simulink model "fmcw_chirp_rom_test"  (R2025b)
settings: Solver=FixedStepDiscrete  StartTime=0.0  StopTime=1.024e-05  FixedStep=5e-09  RelTol=1e-3
libraries: simulink x1
settings Model: DataTypeOverride=Off  Creator=kimsteph  LastModifiedBy=kimsteph
settings OptimizationCC: BlockReduction=off  ConditionallyExecuteInputs=off  DefaultParameterBehavior=Inlined  InheritOutputTypeSmallerThanSingle=on
settings DebuggingCC: ArtificialAlgebraicLoopMsg=error  SingleTaskRateTransMsg=error
settings HardwareCC: ProdBitPerPointer=32.0  ProdBitPerSizeT=32.0  ProdBitPerPtrDiffT=32.0  ProdLargestAtomicFloat=None  ProdIntDivRoundTo=Undefined  ProdEndianess=Unspecified  ProdWordSize=32.0  ProdHWDeviceType=ASIC/FPGA->ASIC/FPGA  TargetBitPerPointer=64.0  TargetBitPerSizeT=64.0  TargetBitPerPtrDiffT=64.0  TargetLongLongMode=on  TargetIntDivRoundTo=Zero  TargetEndianess=LittleEndian  TargetWordSize=64.0  TargetHWDeviceType=Custom Processor->MATLAB Host Computer  ProdEqTarget=off

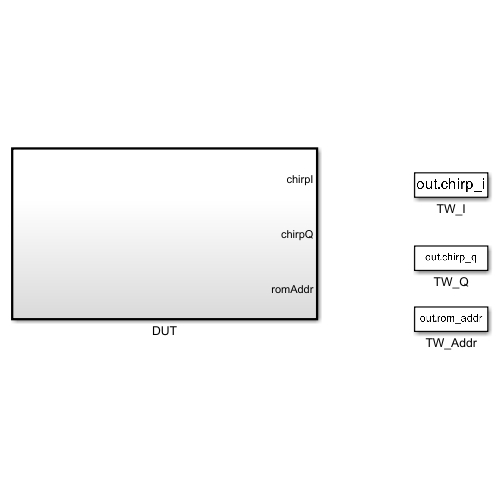
[thumbnail: Simulink's stored preview of the top-level diagram]
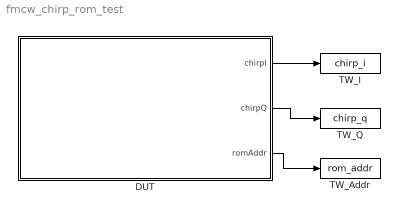
== system fmcw_chirp_rom_test ==
  DUT : Subsystem  TreatAsAtomicUnit=on
  TW_Addr : ToWorkspace  VariableName=rom_addr  SaveFormat=Timeseries  SampleTime=-1
  TW_I : ToWorkspace  VariableName=chirp_i  SaveFormat=Timeseries  SampleTime=-1
  TW_Q : ToWorkspace  VariableName=chirp_q  SaveFormat=Timeseries  SampleTime=-1
  wires:
  DUT/2(chirpQ) -> TW_Q/1
  DUT/1(chirpI) -> TW_I/1
  DUT/3(romAddr) -> TW_Addr/1

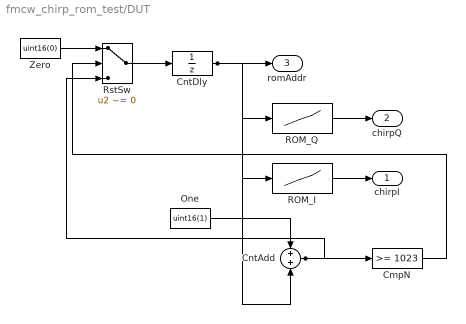
== system fmcw_chirp_rom_test/DUT ==
  CmpN : simulink/Logic and Bit Operations/Compare To Constant  relop=>=  const=1023  OutDataTypeStr=boolean
  CntAdd : Sum  OutDataTypeStr=uint16
  CntDly : UnitDelay  SampleTime=5e-09  HasFrameUpgradeWarning=on
  One : Constant  Value=uint16(1)  OutDataTypeStr=uint16
  ROM_I : Lookup_n-D  NumberOfTableDimensions=1  BreakpointsForDimension1=[0 1 2 3 4 5 6 7 8 9 10 11 12 13 14 15 16 17 18 19 20 21 22 23 24 25 26 27 28 29 30 31 32 33 34 35 36 37 38 39 40 41 42 43 44 45 46 47 48 49 50 51 52 53 54 55 56 57 58 59 60 61 62 63 64 65 66 67 68 69 70 71 72 73 74 75 76 77 78 79 80 81 82 83 84 85 86 87 88 89 90 91 92 93 94 95 96 97 98 99 100 101 102 103 104 105 106 107 108 109 110 111 112 113 114 115 116 117 118 119 120 121 122 123 124 125 126 127 128 129 130 131 132 133 134 135 136 137 138 139 140 141 142 143 144 145 146 147 148 149 150 151 152 153 154 155 156 157 158 159 160 161 162 163 164 165 166 167 168 169 170 171 172 173 174 175 176 177 178 179 180 181 182 183 184 185 186 187 188 189 190 191 192 193 194 195 196 197 198 199 200 201 202 203 204 205 206 207 208 209 210 211 212 213 214 215 216 217 218 219 220 221 222 223 224 225 226 227 228 229 230 231 232 233 234 235 236 237 238 239 240 241 242 243 244 245 246 247 248 249 250 251 252 253 254 255 256 257 258 259 260 261 262 263 264 265 266 267 268 269 270 271 272 273 274 275 276 277 278 279 280 281 282 283 284 285 286 287 288 289 290 291 292 293 294 295 296 297 298 299 300 301 302 303 304 305 306 307 308 309 310 311 312 313 314 315 316 317 318 319 320 321 322 323 324 325 326 327 328 329 330 331 332 333 334 335 336 337 338 339 340 341 342 343 344 345 346 347 348 349 350 351 352 353 354 355 356 357 358 359 360 361 362 363 364 365 366 367 368 369 370 371 372 373 374 375 376 377 378 379 380 381 382 383 384 385 386 387 388 389 390 391 392 393 394 395 396 397 398 399 400 401 402 403 404 405 406 407 408 409 410 411 412 413 414 415 416 417 418 419 420 421 422 423 424 425 426 427 428 429 430 431 432 433 434 435 436 437 438 439 440 441 442 443 444 445 446 447 448 449 450 451 452 453 454 455 456 457 458 459 460 461 462 463 464 465 466 467 468 469 470 471 472 473 474 475 476 477 478 479 480 481 482 483 484 485 486 487 488 489 490 491 492 493 494 495 496 497 498 499 500 501 502 503 504 505 506 507 508 509 510 511 512 513 514 515 516 517 518 519 520 521 522 523 524 525 526 527 528 529 530 531 532 533 534 535 536 537 538 539 540 541 542 543 544 545 546 547 548 549 550 551 552 553 554 555 556 557 558 559 560 561 562 563 564 565 566 567 568 569 570 571 572 573 574 575 576 577 578 579 580 581 582 583 584 585 586 587 588 589 590 591 592 593 594 595 596 597 598 599 600 601 602 603 604 605 606 607 608 609 610 611 612 613 614 615 616 617 618 619 620 621 622 623 624 625 626 627 628 629 630 631 632 633 634 635 636 637 638 639 640 641 642 643 644 645 646 647 648 649 650 651 652 653 654 655 656 657 658 659 660 661 662 663 664 665 666 667 668 669 670 671 672 673 674 675 676 677 678 679 680 681 682 683 684 685 686 687 688 689 690 691 692 693 694 695 696 697 698 699 700 701 702 703 704 705 706 707 708 709 710 711 712 713 714 715 716 717 718 719 720 721 722 723 724 725 726 727 728 729 730 731 732 733 734 735 736 737 738 739 740 741 742 743 744 745 746 747 748 749 750 751 752 753 754 755 756 757 758 759 760 761 762 763 764 765 766 767 768 769 770 771 772 773 774 775 776 777 778 779 780 781 782 783 784 785 786 787 788 789 790 791 792 793 794 795 796 797 798 799 800 801 802 803 804 805 806 807 808 809 810 811 812 813 814 815 816 817 818 819 820 821 822 823 824 825 826 827 828 829 830 831 832 833 834 835 836 837 838 839 840 841 842 843 844 845 846 847 848 849 850 851 852 853 854 855 856 857 858 859 860 861 862 863 864 865 866 867 868 869 870 871 872 873 874 875 876 877 878 879 880 881 882 883 884 885 886 887 888 889 890 891 892 893 894 895 896 897 898 899 900 901 902 903 904 905 906 907 908 909 910 911 912 913 914 915 916 917 918 919 920 921 922 923 924 925 926 927 928 929 930 931 932 933 934 935 936 937 938 939 940 941 942 943 944 945 946 947 948 949 950 951 952 953 954 955 956 957 958 959 960 961 962 963 964 965 966 967 968 969 970 971 972 973 974 975 976 977 978 979 980 981 982 983 984 985 986 987 988 989 990 991 992 993 994 995 996 997 998 999 1000 1001 1002 1003 1004 1005 1006 1007 1008 1009 1010 1011 1012 1013 1014 1015 1016 1017 1018 1019 1020 1021 1022 1023]  Table=[1;0.999999;0.999981;0.999905;0.999699;0.999265;0.998476;0.997176;0.995185;0.992291;0.988258;0.982824;0.975702;0.966584;0.955141;0.941026;0.92388;0.903332;0.879012;0.850549;0.817585;0.779778;0.736817;0.688429;0.634393;0.574553;0.50883;0.437237;0.359895;0.277046;0.189069;0.0964904;-1.60812e-16;-0.0995436;-0.201105;-0.303468;-0.405241;-0.504863;-0.600616;-0.690651;-0.77301;-0.845673;-0.906596;-0.953768;-0.985278;-0.999378;-0.994565;-0.969657;-0.92388;-0.856939;-0.769103;-0.661266;-0.534998;-0.392582;-0.237024;-0.0720347;0.0980171;0.268191;0.433094;0.58704;0.724247;0.83906;0.92621;0.981083;1;0.980485;0.921514;0.823721;0.689541;0.523283;0.331106;0.120888;-0.0980171;-0.315138;-0.519356;-0.699473;-0.844854;-0.946105;-0.995767;-0.98895;-0.92388;-0.802293;-0.629638;-0.415034;-0.170962;0.0873255;0.342661;0.577062;0.77301;0.91483;0.990058;0.990695;0.91421;0.764179;0.550458;0.288816;2.32745e-15;-0.291752;-0.560662;-0.781695;-0.932993;-0.998211;-0.968522;-0.844032;-0.634393;-0.358463;-0.0429383;0.279993;0.575808;0.811355;0.958703;0.998719;0.92388;0.73992;0.465976;0.133061;-0.219101;-0.54661;-0.806848;-0.964184;-0.995185;-0.892534;-0.667;-0.34698;0.0245412;0.395401;0.711432;0.924465;1;0.923291;0.702755;0.369892;-0.0245412;-0.417824;-0.745058;-0.950008;-0.995185;-0.86933;-0.59076;-0.20561;0.219101;0.606731;0.884797;0.99887;0.92388;0.670422;0.284408;-0.160372;-0.575808;-0.876809;-0.999078;-0.913587;-0.634393;-0.217604;0.248928;0.663564;0.932993;0.993737;0.828045;0.470043;6.85988e-15;-0.472749;-0.834863;-0.996443;-0.91421;-0.60429;-0.140658;0.361326;0.77301;0.985539;0.939459;0.642657;0.170962;-0.349856;-0.776888;-0.9894;-0.92388;-0.594466;-0.091909;0.439994;0.844854;0.999942;0.854558;0.448241;-0.0980171;-0.61644;-0.943593;-0.972584;-0.689541;-0.181532;0.388345;0.832321;1;0.830616;0.377007;-0.208612;-0.724247;-0.987544;-0.901349;-0.491563;0.0980171;0.654334;0.971504;0.927935;0.534998;-0.0628518;-0.639124;-0.970403;-0.92388;-0.512786;0.104122;0.681724;0.985278;0.886932;0.422;-0.220598;-0.77301;-0.999735;-0.799537;-0.253382;0.405241;0.888345;0.97957;0.633207;-5.8814e-15;-0.635578;-0.981964;-0.875329;-0.359895;0.32676;0.860867;0.985014;0.634393;-0.0260747;-0.676093;-0.994075;-0.817585;-0.229565;0.476799;0.94206;0.92388;0.426168;-0.296151;-0.864744;-0.975702;-0.564466;0.152797;0.789289;0.995185;0.652011;-0.0551952;-0.733697;-0.999699;-0.697278;0.00613588;0.708191;1;0.706021;-0.00613588;-0.716801;-0.999699;-0.679476;0.0551952;0.75821;0.995185;0.614022;-0.152797;-0.825456;-0.975702;-0.502212;0.296151;0.904644;0.92388;0.335445;-0.476799;-0.973293;-0.817585;-0.108697;0.676093;0.99966;0.634393;-0.172473;-0.860867;-0.945107;-0.359895;0.483527;0.981964;0.772036;1.02889e-14;-0.773983;-0.97957;-0.459177;0.405241;0.967366;0.799537;0.0230077;-0.77301;-0.975365;-0.422;0.4619;0.985278;0.731609;-0.104122;-0.858516;-0.92388;-0.241492;0.639124;0.998023;0.534998;-0.372741;-0.971504;-0.756206;0.0980171;0.870842;0.901349;0.157343;-0.724247;-0.977999;-0.377007;0.556845;1;0.554294;-0.388345;-0.983385;-0.689541;0.23255;0.943593;0.787402;-0.0980171;-0.893913;-0.854558;-0.0107377;0.844854;0.898001;0.091909;-0.80412;-0.92388;-0.145213;0.776888;0.936803;0.170962;-0.766154;-0.939459;-0.16945;0.77301;0.93244;0.140658;-0.796765;-0.91421;-0.0842689;0.834863;0.881197;-2.98944e-14;-0.882643;-0.828045;0.111747;0.932993;0.748119;-0.248928;-0.976037;-0.634393;0.406643;0.999078;0.480839;-0.575808;-0.987057;-0.284408;0.74198;0.92388;0.0475355;-0.884797;-0.794907;0.219101;0.978634;0.59076;-0.494232;-0.995185;-0.312225;0.745058;0.908528;-0.0245412;-0.929075;-0.702755;0.3841;1;0.381266;-0.711432;-0.918508;0.0245412;0.937872;0.667;-0.450981;-0.995185;-0.265234;0.806848;0.837387;-0.219101;-0.991108;-0.465976;0.672695;0.92388;-0.0505997;-0.958703;-0.584554;0.575808;0.960002;0.0429383;-0.933544;-0.634393;0.536293;0.968522;0.0597896;-0.932993;-0.623661;0.560662;0.956494;1.46648e-15;-0.957385;-0.550458;0.645005;0.91421;-0.136101;-0.990058;-0.403838;0.77301;0.816701;-0.342661;-0.99618 ...(+5587 chars)]  InterpMethod=Flat  InternalRulePriority=Speed  OutDataTypeStr=fixdt(1,16,14)  RndMeth=Simplest
  ROM_Q : Lookup_n-D  NumberOfTableDimensions=1  BreakpointsForDimension1=[0 1 2 3 4 5 6 7 8 9 10 11 12 13 14 15 16 17 18 19 20 21 22 23 24 25 26 27 28 29 30 31 32 33 34 35 36 37 38 39 40 41 42 43 44 45 46 47 48 49 50 51 52 53 54 55 56 57 58 59 60 61 62 63 64 65 66 67 68 69 70 71 72 73 74 75 76 77 78 79 80 81 82 83 84 85 86 87 88 89 90 91 92 93 94 95 96 97 98 99 100 101 102 103 104 105 106 107 108 109 110 111 112 113 114 115 116 117 118 119 120 121 122 123 124 125 126 127 128 129 130 131 132 133 134 135 136 137 138 139 140 141 142 143 144 145 146 147 148 149 150 151 152 153 154 155 156 157 158 159 160 161 162 163 164 165 166 167 168 169 170 171 172 173 174 175 176 177 178 179 180 181 182 183 184 185 186 187 188 189 190 191 192 193 194 195 196 197 198 199 200 201 202 203 204 205 206 207 208 209 210 211 212 213 214 215 216 217 218 219 220 221 222 223 224 225 226 227 228 229 230 231 232 233 234 235 236 237 238 239 240 241 242 243 244 245 246 247 248 249 250 251 252 253 254 255 256 257 258 259 260 261 262 263 264 265 266 267 268 269 270 271 272 273 274 275 276 277 278 279 280 281 282 283 284 285 286 287 288 289 290 291 292 293 294 295 296 297 298 299 300 301 302 303 304 305 306 307 308 309 310 311 312 313 314 315 316 317 318 319 320 321 322 323 324 325 326 327 328 329 330 331 332 333 334 335 336 337 338 339 340 341 342 343 344 345 346 347 348 349 350 351 352 353 354 355 356 357 358 359 360 361 362 363 364 365 366 367 368 369 370 371 372 373 374 375 376 377 378 379 380 381 382 383 384 385 386 387 388 389 390 391 392 393 394 395 396 397 398 399 400 401 402 403 404 405 406 407 408 409 410 411 412 413 414 415 416 417 418 419 420 421 422 423 424 425 426 427 428 429 430 431 432 433 434 435 436 437 438 439 440 441 442 443 444 445 446 447 448 449 450 451 452 453 454 455 456 457 458 459 460 461 462 463 464 465 466 467 468 469 470 471 472 473 474 475 476 477 478 479 480 481 482 483 484 485 486 487 488 489 490 491 492 493 494 495 496 497 498 499 500 501 502 503 504 505 506 507 508 509 510 511 512 513 514 515 516 517 518 519 520 521 522 523 524 525 526 527 528 529 530 531 532 533 534 535 536 537 538 539 540 541 542 543 544 545 546 547 548 549 550 551 552 553 554 555 556 557 558 559 560 561 562 563 564 565 566 567 568 569 570 571 572 573 574 575 576 577 578 579 580 581 582 583 584 585 586 587 588 589 590 591 592 593 594 595 596 597 598 599 600 601 602 603 604 605 606 607 608 609 610 611 612 613 614 615 616 617 618 619 620 621 622 623 624 625 626 627 628 629 630 631 632 633 634 635 636 637 638 639 640 641 642 643 644 645 646 647 648 649 650 651 652 653 654 655 656 657 658 659 660 661 662 663 664 665 666 667 668 669 670 671 672 673 674 675 676 677 678 679 680 681 682 683 684 685 686 687 688 689 690 691 692 693 694 695 696 697 698 699 700 701 702 703 704 705 706 707 708 709 710 711 712 713 714 715 716 717 718 719 720 721 722 723 724 725 726 727 728 729 730 731 732 733 734 735 736 737 738 739 740 741 742 743 744 745 746 747 748 749 750 751 752 753 754 755 756 757 758 759 760 761 762 763 764 765 766 767 768 769 770 771 772 773 774 775 776 777 778 779 780 781 782 783 784 785 786 787 788 789 790 791 792 793 794 795 796 797 798 799 800 801 802 803 804 805 806 807 808 809 810 811 812 813 814 815 816 817 818 819 820 821 822 823 824 825 826 827 828 829 830 831 832 833 834 835 836 837 838 839 840 841 842 843 844 845 846 847 848 849 850 851 852 853 854 855 856 857 858 859 860 861 862 863 864 865 866 867 868 869 870 871 872 873 874 875 876 877 878 879 880 881 882 883 884 885 886 887 888 889 890 891 892 893 894 895 896 897 898 899 900 901 902 903 904 905 906 907 908 909 910 911 912 913 914 915 916 917 918 919 920 921 922 923 924 925 926 927 928 929 930 931 932 933 934 935 936 937 938 939 940 941 942 943 944 945 946 947 948 949 950 951 952 953 954 955 956 957 958 959 960 961 962 963 964 965 966 967 968 969 970 971 972 973 974 975 976 977 978 979 980 981 982 983 984 985 986 987 988 989 990 991 992 993 994 995 996 997 998 999 1000 1001 1002 1003 1004 1005 1006 1007 1008 1009 1010 1011 1012 1013 1014 1015 1016 1017 1018 1019 1020 1021 1022 1023]  Table=[0;0.00153398;0.00613588;0.0138054;0.0245412;0.0383401;0.0551952;0.0750943;0.0980171;0.123933;0.152797;0.184548;0.219101;0.256349;0.296151;0.338334;0.382683;0.428941;0.476799;0.525895;0.575808;0.626056;0.676093;0.725304;0.77301;0.818467;0.860867;0.899346;0.932993;0.960857;0.981964;0.995334;1;0.995033;0.97957;0.952842;0.91421;0.863199;0.799537;0.723188;0.634393;0.533701;0.422;0.300543;0.170962;0.0352742;-0.104122;-0.244468;-0.382683;-0.515418;-0.639124;-0.750152;-0.844854;-0.919717;-0.971504;-0.997402;-0.995185;-0.963366;-0.901349;-0.809558;-0.689541;-0.544039;-0.377007;-0.193586;6.43249e-16;0.196595;0.388345;0.566996;0.724247;0.852159;0.943593;0.992666;0.995185;0.949046;0.854558;0.714659;0.534998;0.323859;0.091909;-0.148248;-0.382683;-0.596931;-0.776888;-0.909806;-0.985278;-0.99618;-0.939459;-0.816701;-0.634393;-0.403838;-0.140658;0.136101;0.405241;0.645005;0.834863;0.957385;1;0.956494;0.828045;0.623661;0.359895;0.0597896;-0.248928;-0.536293;-0.77301;-0.933544;-0.999078;-0.960002;-0.817585;-0.584554;-0.284408;0.0505997;0.382683;0.672695;0.884797;0.991108;0.975702;0.837387;0.59076;0.265234;-0.0980171;-0.450981;-0.745058;-0.937872;-0.999699;-0.918508;-0.702755;-0.381266;2.573e-15;0.3841;0.711432;0.929075;0.999699;0.908528;0.667;0.312225;-0.0980171;-0.494232;-0.806848;-0.978634;-0.975702;-0.794907;-0.465976;-0.0475355;0.382683;0.74198;0.958703;0.987057;0.817585;0.480839;0.0429383;-0.406643;-0.77301;-0.976037;-0.968522;-0.748119;-0.359895;0.111747;0.560662;0.882643;1;0.881197;0.550458;0.0842689;-0.405241;-0.796765;-0.990058;-0.93244;-0.634393;-0.16945;0.342661;0.766154;0.985278;0.936803;0.629638;0.145213;-0.382683;-0.80412;-0.995767;-0.898001;-0.534998;-0.0107377;0.519356;0.893913;0.995185;0.787402;0.331106;-0.23255;-0.724247;-0.983385;-0.921514;-0.554294;-9.30979e-15;0.556845;0.92621;0.977999;0.689541;0.157343;-0.433094;-0.870842;-0.995185;-0.756206;-0.237024;0.372741;0.844854;0.998023;0.769103;0.241492;-0.382683;-0.858516;-0.994565;-0.731609;-0.170962;0.4619;0.906596;0.975365;0.634393;0.0230077;-0.600616;-0.967366;-0.91421;-0.459177;0.201105;0.773983;1;0.772036;0.189069;-0.483527;-0.932993;-0.945107;-0.50883;0.172473;0.77301;0.99966;0.736817;0.108697;-0.575808;-0.973293;-0.879012;-0.335445;0.382683;0.904644;0.955141;0.502212;-0.219101;-0.825456;-0.988258;-0.614022;0.0980171;0.75821;0.998476;0.679476;-0.0245412;-0.716801;-0.999981;-0.706021;1.0292e-14;0.708191;0.999981;0.697278;-0.0245412;-0.733697;-0.998476;-0.652011;0.0980171;0.789289;0.988258;0.564466;-0.219101;-0.864744;-0.955141;-0.426168;0.382683;0.94206;0.879012;0.229565;-0.575808;-0.994075;-0.736817;0.0260747;0.77301;0.985014;0.50883;-0.32676;-0.932993;-0.875329;-0.189069;0.635578;1;0.633207;-0.201105;-0.888345;-0.91421;-0.253382;0.600616;0.999735;0.634393;-0.220598;-0.906596;-0.886932;-0.170962;0.681724;0.994565;0.512786;-0.382683;-0.970403;-0.769103;0.0628518;0.844854;0.927935;0.237024;-0.654334;-0.995185;-0.491563;0.433094;0.987544;0.689541;-0.208612;-0.92621;-0.830616;-2.74395e-14;0.832321;0.921514;0.181532;-0.724247;-0.972584;-0.331106;0.61644;0.995185;0.448241;-0.519356;-0.999942;-0.534998;0.439994;0.995767;0.594466;-0.382683;-0.9894;-0.629638;0.349856;0.985278;0.642657;-0.342661;-0.985539;-0.634393;0.361326;0.990058;0.60429;-0.405241;-0.996443;-0.550458;0.472749;1;0.470043;-0.560662;-0.993737;-0.359895;0.663564;0.968522;0.217604;-0.77301;-0.913587;-0.0429383;0.876809;0.817585;-0.160372;-0.958703;-0.670422;0.382683;0.99887;0.465976;-0.606731;-0.975702;-0.20561;0.806848;0.86933;-0.0980171;-0.950008;-0.667;0.417824;0.999699;0.369892;-0.711432;-0.923291;-3.72392e-14;0.924465;0.702755;-0.395401;-0.999699;-0.34698;0.745058;0.892534;-0.0980171;-0.964184;-0.59076;0.54661;0.975702;0.133061;-0.884797;-0.73992;0.382683;0.998719;0.284408;-0.811355;-0.817585;0.279993;0.999078;0.358463;-0.77301;-0.844032;0.248928;0.998211;0.359895;-0.781695;-0.828045;0.291752;1;0.288816;-0.834863;-0.764179;0.405241;0.990695;0.140658;-0.91483;-0.634393;0.577062;0.939459;-0.0873255;-0.985278 ...(+5605 chars)]  InterpMethod=Flat  InternalRulePriority=Speed  OutDataTypeStr=fixdt(1,16,14)  RndMeth=Simplest
  RstSw : Switch  Criteria=u2 ~= 0  SaturateOnIntegerOverflow=off  InputSameDT=off
  Zero : Constant  Value=uint16(0)  OutDataTypeStr=uint16
  chirpI : Outport
  chirpQ : Outport  Port=2
  romAddr : Outport  Port=3
  wires:
  ROM_Q/1 -> chirpQ/1
  Zero/1 -> RstSw/1
  RstSw/1 -> CntDly/1
  CntAdd/1 -> CmpN/1, RstSw/3
  CntDly/1 -> ROM_Q/1, romAddr/1, ROM_I/1, CntAdd/2
  ROM_I/1 -> chirpI/1
  One/1 -> CntAdd/1
  CmpN/1 -> RstSw/2
